simulink model "DS_distrIntp_1_10_simulated axes"  (R2019a)
settings: Solver=FixedStepDiscrete  StartTime=0.0  StopTime=inf  FixedStep=Ts  RelTol=1e-3
InitFcn:
  | %% Verwende vordefinierte Setpoints (Kreis mit Z-Komponente)
  | 
  | % Config
  | numCircles = 3;
  | scale=6;
  | %Versuch symmetrische Setpunkte zu setzen
  | pointsPerCircle =scale*(4+3*numCircles)+2;
  | 
  | r = 50;
  | m_x = r;
  | m_y = r;
  | 
  | % //
  | s = linspace(0,2*pi,pointsPerCircle);
  | 
  | setPoints_x = [];
  | setPoints_y = [];
  | 
  | for ii=1:numCircles
  | 
  | setPoints_x = [setPoints_x (-cos(s(1:floor(pointsPerCircle / 2))).*r + m_x + 2*r*(ii-1))]; %#ok<AGROW>
  | setPoints_y = [setPoints_y (sin(s).*r+m_y)]; %#ok<AGROW>pointsPerCircle / 2
  | 
  | end
  | 
  | setPoints_x = [setPoints_x flip(setPoints_x(1:end))];
  | 
  | % Loeschen doppelter y-Werte (Kreisuebergang)
  | setPoints_x(pointsPerCircle .* [1:numCircles]) = [];
  | setPoints_y(pointsPerCircle .* [1:numCircles]) = [];
  | 
  | % setPoints_x= [linspace(0,setPoints_x(19),19) setPoints_x(20:end)];
  | % setPoints_y= [linspace(0,setPoints_y(19),19) setPoints_y(20:end)];
  | 
  | % Array Elemente verschieben
  | % setPoints_x = circshift(setPoints_x,-pointsPerCircle/4,2);
  | % setPoints_y = circshift(setPoints_y,-pointsPerCircle/4,2);
  | 
  | z = zeros(1,size(setPoints_x,2));
  | z_x = -5:5;
  | z_y = -z_x.^2 + 25;
  | z_idx = 90;
  | z_idx2 = 210;
  | z(z_idx:z_idx+length(z_x)-1) = z_y;
  | z(z_idx2:z_idx2+length(z_x)-1) = z_y;
  | % z = [z_y z];
  | setPoints_z = z;
  | 
  | % setPoints_x = [zeros(1,length(z_y)) setPoints_x];
  | % setPoints_y = [setPoints_y(1,1)*ones(1,length(z_y)) setPoints_y];
  | 
  | % Umrechnung der Einheiten für Demonstrator
  | % setPoints_x = setPoints_x ./ 1000;
  | % setPoints_y = setPoints_y ./ 1000;
  | % setPoints_z = setPoints_z ./ 1000;
  | 
  | 
  | %{
  | plot(setPoints_x,setPoints_y);
  | fig = figure;
  | plot3(setPoints_x(1:end-1),setPoints_y(1:end-1),setPoints_z(1:end-1));
  | 
  | ax = gca;
  | ax.YDir = 'reverse';
  | ax.ZDir = 'reverse';
  | %}
  | 
  | % setPoints_z = zeros(1,size(setPoints_x,2));
  | 
  | setP_mat = [setPoints_x;setPoints_y;setPoints_z];
  | %Dauerlauftest zehn Durchgänge
  | %setP_mat = repmat(setP_mat, 1, 10);
  | setP_mat = setP_mat(:,2:end);
StartFcn:
  | close all;
model workspace (MAT data in the model file):
  MvmtPerfEval_collectVal = Simulink.Parameter
  MvmtPerfEval_collectVal.Value = 0.65
  MvmtPerfEval_collectVal.Description = '- Anteil eines Interpolationssegments (0,1)
    | - Nach Abarbeitung des spezifizierten Anteils wird gemeinsame Performance aller Agenten
    | vom Dispatcher geladen
    | 
    | - (!!!) Wert MUSS größer sein als MvmtPerfEval_sendOwnVal'
  MvmtPerfEval_collectVal.DataType = 'auto'
  MvmtPerfEval_collectVal.Min = 0
  MvmtPerfEval_collectVal.Max = 1
  MvmtPerfEval_collectVal.Dimensions = [1 1]
  MvmtPerfEval_sendOwnVal = Simulink.Parameter
  MvmtPerfEval_sendOwnVal.Value = 0.6
  MvmtPerfEval_sendOwnVal.Description = '- Anteil eines Interpolationssegments (0,1)
    | - Nach Abarbeitung des spezifizierten Anteils wird Perfomance Kennzahl an Dispatcher übermittelt
    | 
    | - (!!!) Wert MUSS kleiner sein als MvmtPerfEval_collectVal'
  MvmtPerfEval_sendOwnVal.DataType = 'auto'
  MvmtPerfEval_sendOwnVal.Min = 0
  MvmtPerfEval_sendOwnVal.Max = 1
  MvmtPerfEval_sendOwnVal.Dimensions = [1 1]
  PerfEval_numTicks_enable = Simulink.Parameter
  PerfEval_numTicks_enable.Value = 10
  PerfEval_numTicks_enable.Description = 'Anzahl der Ticks (Integrationsschritte), bevor die Performance ausgewertet wird
    | (unabhängig vom Senden des Werts an den Dispatcher)'
  PerfEval_numTicks_enable.DataType = 'auto'
  PerfEval_numTicks_enable.Dimensions = [1 1]
  Segmentregler_I_Gain = Simulink.Parameter
  Segmentregler_I_Gain.Value = 1
  Segmentregler_I_Gain.DataType = 'auto'
  Segmentregler_I_Gain.Dimensions = [1 1]
  Segmentregler_P_Gain = Simulink.Parameter
  Segmentregler_P_Gain.Value = 0
  Segmentregler_P_Gain.DataType = 'auto'
  Segmentregler_P_Gain.Dimensions = [1 1]
  Segmentregler_minVel_enable = Simulink.Parameter
  Segmentregler_minVel_enable.Value = 0.1
  Segmentregler_minVel_enable.DataType = 'auto'
  Segmentregler_minVel_enable.Dimensions = [1 1]
  Segmentregler_numTicks_enable = Simulink.Parameter
  Segmentregler_numTicks_enable.Value = 30
  Segmentregler_numTicks_enable.Description = 'Anzahl der Ticks (Integrationsschritte), bevor der Segmentregler aktiv wird'
  Segmentregler_numTicks_enable.DataType = 'auto'
  Segmentregler_numTicks_enable.Dimensions = [1 1]
  Ts = Simulink.Parameter
  Ts.Value = 0.005
  Ts.Description = 'Sampling Time'
  Ts.DataType = 'auto'
  Ts.Dimensions = [1 1]
  maxPos_x = Simulink.Parameter
  maxPos_x.Value = 300
  maxPos_x.Description = 'Grenze des Arbeitsbereichs (maximaler Wert der Koordinate)'
  maxPos_x.DataType = 'auto'
  maxPos_x.Dimensions = [1 1]
  maxPos_y = Simulink.Parameter
  maxPos_y.Value = 150
  maxPos_y.Description = 'Grenze des Arbeitsbereichs (maximaler Wert der Koordinate)'
  maxPos_y.DataType = 'auto'
  maxPos_y.Dimensions = [1 1]
  maxPos_z = Simulink.Parameter
  maxPos_z.Value = 50
  maxPos_z.Description = 'Grenze des Arbeitsbereichs (maximaler Wert der Koordinate)'
  maxPos_z.DataType = 'auto'
  maxPos_z.Dimensions = [1 1]
  maxVectorLengths = Simulink.Parameter
  maxVectorLengths.Value = 100000
  maxVectorLengths.DataType = 'auto'
  maxVectorLengths.Dimensions = [1 1]
  minAllowedVelSaturation = Simulink.Parameter
  minAllowedVelSaturation.Value = 0.05
  minAllowedVelSaturation.Description = 'Minimaler Saturation-Wert für den Geschwindigkeits-PID-Regler
    | (auch bei Sollgeschwindigkeit soll Fehlerkorrektur möglich sein)'
  minAllowedVelSaturation.DataType = 'auto'
  minAllowedVelSaturation.Dimensions = [1 1]
  numAxes = Simulink.Parameter
  numAxes.Value = 3
  numAxes.DataType = 'auto'
  numAxes.Dimensions = [1 1]
undefined symbols (not defined in the file or in its folder): DiscIntNeverNeededParam, VelOverride
libraries: simulink x19, vrlib x5, sldrtlib x2
(part 1 of 4)
settings Model: EnablePacing=on  PacingRate=10  Creator=Daniel  LastModifiedBy=Daniel
settings DataIOCC: ReturnWorkspaceOutputs=off
settings DebuggingCC: ArithmeticOperatorsInVariantConditions=warning

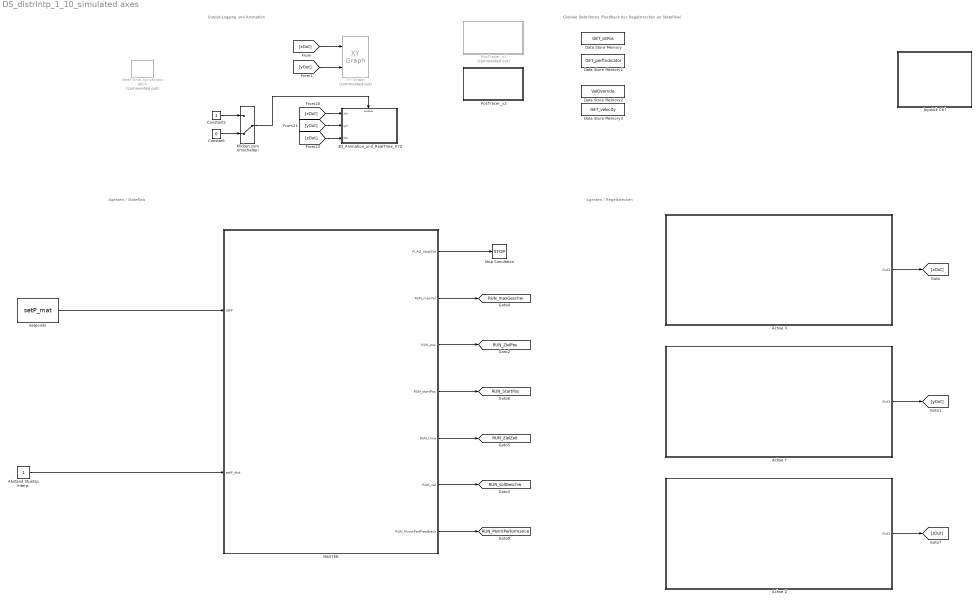
== system DS_distrIntp_1_10_simulated axes ==
  note: Globale DataStores (Feedback der Regelstrecken an Stateflow)
  note: Agenten / Regelstrecken
  note: Agenten / Stateflow
  note: Output-Logging und Animation
  3D_Animation_und_RealTime_XYZ : Subsystem
  Abstand Stuetzp. Interp. : Constant
  Achse X : Subsystem
  Achse Y : Subsystem
  Achse Z : Subsystem
  Constant : Constant  Value=0
  Constant1 : Constant
  Data Store Memory : DataStoreMemory  DataStoreName=GET_istPos  ReadBeforeWriteMsg=warning  WriteAfterWriteMsg=warning  WriteAfterReadMsg=warning  InitialValue=zeros(1,numAxes)  ShowAdditionalParam=off  OutDataTypeStr=double
  Data Store Memory1 : DataStoreMemory  DataStoreName=GET_perfIndicator  ReadBeforeWriteMsg=warning  WriteAfterWriteMsg=warning  WriteAfterReadMsg=warning  InitialValue=zeros(1,numAxes)  ShowAdditionalParam=off  OutDataTypeStr=double
  Data Store Memory2 : DataStoreMemory  DataStoreName=VelOverride  ReadBeforeWriteMsg=warning  WriteAfterWriteMsg=warning  WriteAfterReadMsg=warning  InitialValue=ones(1,numAxes)  ShowAdditionalParam=off  OutDataTypeStr=double
  Data Store Memory3 : DataStoreMemory  DataStoreName=GET_velocity  ReadBeforeWriteMsg=warning  WriteAfterWriteMsg=warning  WriteAfterReadMsg=warning  InitialValue=zeros(1,numAxes)  ShowAdditionalParam=off  OutDataTypeStr=double
  Joystick Ctrl : Subsystem
  Klicken zum Umschalten : ManualSwitch  CurrentSetting=0
  MASTER : Stateflow chart  TreatAsAtomicUnit=on
  PosTracer_v1 : Stateflow chart  Commented=on  BlockKeywords=__PRM__SERIALIZED__DATA__:Stateflow Chart,Stateflow Diagram  TreatAsAtomicUnit=on
  PosTracer_v2 : Stateflow chart  BlockKeywords=__PRM__SERIALIZED__DATA__:Stateflow Chart,Stateflow Diagram  TreatAsAtomicUnit=on
  Real-Time Synchronization : sldrtlib/Real-Time Synchronization  Commented=on  SampleTime=0.005  MaxMissedTicks=1000  ShowMissedTicks=off  YieldWhenWaiting=off
  Setpoints : Constant  Value=setP_mat
  Stop Simulation : Stop
  XY Graph : simulink/Sinks/XY Graph  Commented=on  xmin=0  xmax=maxPos_x  ymin=0  ymax=maxPos_y  st=-1
  tag scope: RUN_MvmtPerformance=global, RUN_StartPos=global, RUN_ZielPos=global, RUN_ZielZeit=global, RUN_maxGeschw=global, RUN_sollGeschw=global
  wires:
  Abstand Stuetzp. Interp./1 -> MASTER/2(setP_dist)
  Setpoints/1 -> MASTER/1(setP)
  Achse X/1(Out1) -> [xOut]
  [xOut] -> XY Graph/1
  [yOut] -> XY Graph/2
  Constant/1 -> Klicken zum Umschalten/2
  Constant1/1 -> Klicken zum Umschalten/1
  [xOut] -> 3D_Animation_und_RealTime_XYZ/1(xIn)
  [yOut] -> 3D_Animation_und_RealTime_XYZ/2(yIn)
  [zOut] -> 3D_Animation_und_RealTime_XYZ/3(zIn)
  MASTER/1(FLAG_stopSim) -> Stop Simulation/1
  MASTER/2(RUN_maxVel) -> [RUN_maxGeschw]
  MASTER/3(RUN_pos) -> [RUN_ZielPos]
  MASTER/4(RUN_startPos) -> [RUN_StartPos]
  MASTER/5(RUN_time) -> [RUN_ZielZeit]
  MASTER/6(RUN_vel) -> [RUN_sollGeschw]
  Achse Y/1(Out1) -> [yOut]
  Achse Z/1(Out1) -> [zOut]
  Klicken zum Umschalten/1 -> 3D_Animation_und_RealTime_XYZ/Enable
  MASTER/7(RUN_MvmtPerfFeedback) -> [RUN_MvmtPerformance]

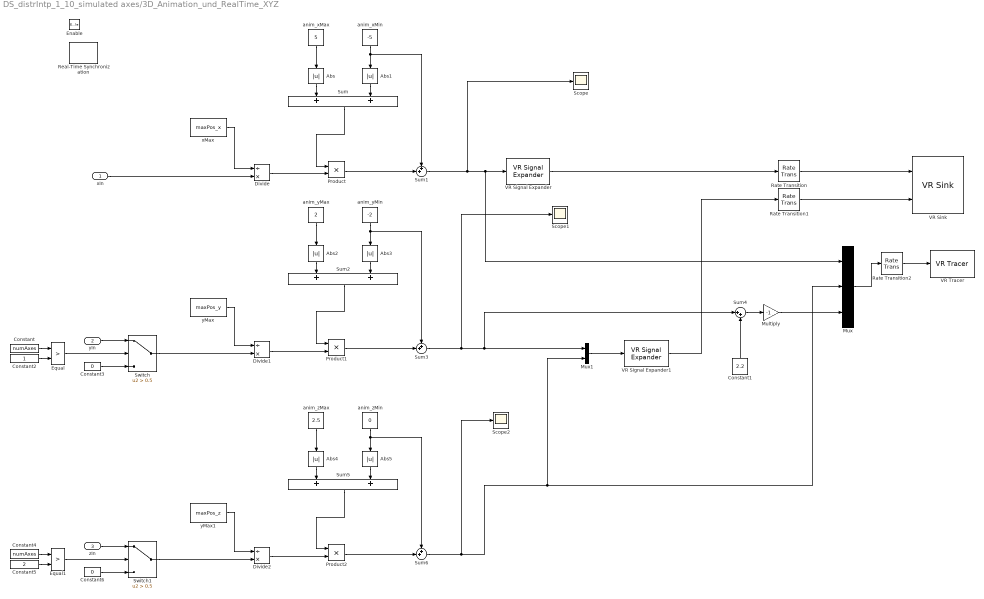
== system DS_distrIntp_1_10_simulated axes/3D_Animation_und_RealTime_XYZ ==
  xIn : Inport
  yIn : Inport  Port=2
  zIn : Inport  Port=3
  Enable : EnablePort
  Abs{,1..5} (6 alike) : Abs
  Constant : Constant  Value=numAxes
  Constant1 : Constant  Value=2.2
  Constant2 : Constant
  Constant3 : Constant  Value=0
  Constant4 : Constant  Value=numAxes
  Constant5 : Constant  Value=2
  Constant6 : Constant  Value=0
  Divide : Product  Inputs=/*
  Divide1 : Product  Inputs=/*
  Divide2 : Product  Inputs=/*
  Equal : RelationalOperator  Operator=>  OutDataTypeStr=boolean  RndMeth=Simplest
  Equal1 : RelationalOperator  Operator=>  OutDataTypeStr=boolean  RndMeth=Simplest
  Multiply : Gain  Gain=-1
  Mux : Mux  Inputs=3
  Mux1 : Mux  Inputs=2
  Product : Product
  Product1 : Product
  Product2 : Product
  Rate Transition : RateTransition  OutPortSampleTime=0.1
  Rate Transition1 : RateTransition  OutPortSampleTime=0.1
  Rate Transition2 : RateTransition  OutPortSampleTime=0.3
  Real-Time Synchronization : sldrtlib/Real-Time Synchronization  SampleTime=0.005  MaxMissedTicks=1000  ShowMissedTicks=off  YieldWhenWaiting=off
  Scope : Scope
  Scope1 : Scope
  Scope2 : Scope
  Sum : Sum
  Sum1 : Sum  Inputs=++|
  Sum2 : Sum
  Sum3 : Sum  Inputs=++|
  Sum4 : Sum  Inputs=|++
  Sum5 : Sum
  Sum6 : Sum  Inputs=++|
  Switch : Switch  Criteria=u2 > Threshold  Threshold=0.5
  Switch1 : Switch  Criteria=u2 > Threshold  Threshold=0.5
  VR Signal Expander : vrlib/VR Signal Expander  outwidth=3  outidx=1
      settings: SourceProductName=Simulink
  VR Signal Expander1 : vrlib/VR Signal Expander  outwidth=3  outidx=[1 2]
      settings: SourceProductName=Simulink
  VR Sink : vrlib/VR Sink  InstantiateOnLoad=on  SampleTime=-1  ViewEnable=on  RemoteChange=off  RemoteView=off  FieldsWritten=yAchse.translation.3.1.1.double#TCP.translation.3.1.1.double  WorldFileName=DS_MA_3dworld.wrl  WorldDescription=DS_MA_3dworld  AutoView=on  VideoDimensions=[]  AllowVariableSize=off  FigureProperties="{'Position', 'Name', 'Viewpoint', 'CameraBound', 'CameraDirection', 'CameraPosition', 'CameraUpVector', 'ZoomFactor', 'Antialiasing', 'Headlight', 'Lighting', 'NavPanel', 'Sound', 'StatusBar', 'Stereo3D', 'Stereo3DCameraOffset', 'Stereo3DHIT', 'ToolBar', 'Textures', 'Transparency', 'Triad', 'Wireframe', 'NavZones', 'NavMode', 'NavSpeed', 'CaptureFileFormat', 'CaptureFileName', 'Record2DCompressMethod', 'Record2DCompressQuality', 'Record2D', 'Record2DFileName', 'Record2DFPS'; [5.0000000000000000e+00   9.2000000000000000e+01   5.7600000000000000e+02   3.5000000000000000e+02], 'DS_MA_3dworld', '_untitled_1', 'on', [0.0000000000000000e+00   0.0000000000000000e+00  -1.0000000000000000e+00], [0.0000000000000000e+00   0.0000000000000000e+00   0.0000000000000000e+00], [0.0000000000000000e+00   1.0000000000000000e+00   0.0000000000000000e+00], [1.0000000000000000e+00], 'on', 'on', 'on', 'halfbar', 'on', 'on', 'off', [1.0000000149011612e-01], [0.0000000000000000e+00], 'on', 'on', 'on', 'none', 'off', 'off', 'fly', 'normal', 'tif', '%f_anim_%n.tif', 'auto', [7.5000000000000000e+01], 'off', '%f_anim_%n.avi', 'auto'}"
      settings: SourceProductName=Simulink
  VR Tracer : vrlib/VR Tracer  VrmlFile=DS_MA_3dworld.wrl  MarkerName=Tetrahedron  UseLines=on  UseTriads=on  MarkerScale=[0.1 0.1 0.1]  MarkerColorSelection=Selected from color list  MarkerColor=red  rgbval=[1 0 0]  Ts=0.3  ForceViewerOpen=off  ConnectPlane=off  PlaneCoeff=[0 1 0 0]  ConnectPoint=None  PointCoord=[0 0 0]
      settings: SourceProductName=Simulink  SourceProductBaseCode=SL
  anim_xMax : Constant  Value=5
  anim_xMin : Constant  Value=-5
  anim_yMax : Constant  Value=2
  anim_yMin : Constant  Value=-2
  anim_zMax : Constant  Value=2.5
  anim_zMin : Constant  Value=0
  xMax : Constant  Value=maxPos_x
  yMax : Constant  Value=maxPos_y
  yMax1 : Constant  Value=maxPos_z
  wires:
  Constant1/1 -> Sum4/2
  Sum4/1 -> Multiply/1
  Multiply/1 -> Mux/3
  Rate Transition2/1 -> VR Tracer/1
  Mux/1 -> Rate Transition2/1
  Rate Transition1/1 -> VR Sink/2
  Rate Transition/1 -> VR Sink/1
  VR Signal Expander/1 -> Rate Transition/1
  VR Signal Expander1/1 -> Rate Transition1/1
  Sum3/1 -> Mux1/1, Sum4/1, Scope1/1
  Sum1/1 -> VR Signal Expander/1, Mux/1, Scope/1
  Switch/1 -> Divide1/2
  yMax/1 -> Divide1/1
  anim_yMax/1 -> Abs2/1
  anim_yMin/1 -> Sum3/1, Abs3/1
  Abs2/1 -> Sum2/1
  Abs3/1 -> Sum2/2
  Divide1/1 -> Product1/2
  Sum2/1 -> Product1/1
  Product1/1 -> Sum3/2
  Product/1 -> Sum1/2
  Sum/1 -> Product/1
  Divide/1 -> Product/2
  Abs1/1 -> Sum/2
  Abs/1 -> Sum/1
  anim_xMin/1 -> Abs1/1, Sum1/1
  anim_xMax/1 -> Abs/1
  xMax/1 -> Divide/1
  xIn/1 -> Divide/2
  Product2/1 -> Sum6/2
  Sum5/1 -> Product2/1
  Divide2/1 -> Product2/2
  Abs5/1 -> Sum5/2
  Abs4/1 -> Sum5/1
  anim_zMin/1 -> Abs5/1, Sum6/1
  anim_zMax/1 -> Abs4/1
  yMax1/1 -> Divide2/1
  Switch1/1 -> Divide2/2
  Sum6/1 -> Scope2/1, Mux1/2, Mux/2
  Mux1/1 -> VR Signal Expander1/1
  Constant/1 -> Equal/1
  Constant2/1 -> Equal/2
  yIn/1 -> Switch/1
  Equal/1 -> Switch/2
  Constant3/1 -> Switch/3
  Constant6/1 -> Switch1/3
  Equal1/1 -> Switch1/2
  zIn/1 -> Switch1/1
  Constant5/1 -> Equal1/2
  Constant4/1 -> Equal1/1

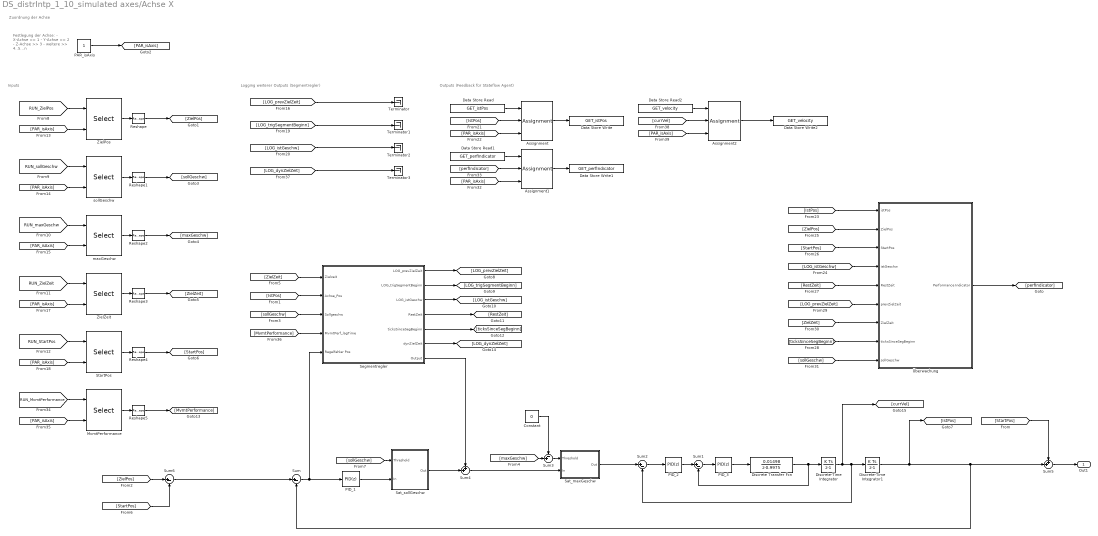
== system DS_distrIntp_1_10_simulated axes/Achse X ==
  note: Outputs (Feedback für Stateflow Agent)
  note: Logging weiterer Outputs (Segmentregler)
  note: Zuordnung der Achse
  note: Festlegung der Achse:
      | - X-Achse >> 1
      | - Y-Achse >> 2
      | - Z-Achse >> 3
      | - weitere >> 4..5...n
  note: Inputs
  Assignment : Assignment  DiagnosticForDimensions=Warning  IndexOptions=Index vector (port)  Indices=1  OutputSizes=1
  Assignment1 : Assignment  DiagnosticForDimensions=Warning  IndexOptions=Index vector (port)  Indices=1  OutputSizes=1
  Assignment2 : Assignment  DiagnosticForDimensions=Warning  IndexOptions=Index vector (port)  Indices=1  OutputSizes=1
  Constant : Constant  Value=0
  Data Store Read : DataStoreRead  DataStoreName=GET_istPos
  Data Store Read1 : DataStoreRead  DataStoreName=GET_perfIndicator
  Data Store Read2 : DataStoreRead  DataStoreName=GET_velocity
  Data Store Write : DataStoreWrite  DataStoreName=GET_istPos
  Data Store Write1 : DataStoreWrite  DataStoreName=GET_perfIndicator
  Data Store Write2 : DataStoreWrite  DataStoreName=GET_velocity
  Discrete Transfer Fcn : DiscreteTransferFcn  Numerator=0.01498  Denominator=[1 -0.9975]
  Discrete-Time Integrator : DiscreteIntegrator  SampleTime=-1  ICPrevOutput=DiscIntNeverNeededParam  ICPrevScaledInput=DiscIntNeverNeededParam
  Discrete-Time Integrator1 : DiscreteIntegrator  SampleTime=-1  ICPrevOutput=DiscIntNeverNeededParam  ICPrevScaledInput=DiscIntNeverNeededParam
  MvmtPerformance : Selector  IndexOptions=Index vector (port)  Indices=[1 3]  OutputSizes=1
  PAR_isAxis : Constant
  PID_1 : simulink/Continuous/PID Controller  Controller=PID  Form=Parallel  TimeDomain=Discrete-time  SampleTime=-1  IntegratorMethod=Forward Euler  FilterMethod=Forward Euler  ControllerParametersSource=internal  P=20  I=0  D=0  UseFilter=on  N=100  TunerSelectOption=Transfer Function Based (PID Tuner App)  InitialConditionSource=internal  InitialConditionForIntegrator=0  InitialConditionForFilter=0  DifferentiatorICPrevScaledInput=0  ExternalReset=none  TrackingMode=off  Kt=1  LimitOutput=off  UpperSaturationLimit=inf  LowerSaturationLimit=-inf  LinearizeAsGain=off  AntiWindupMode=none  Kb=1  POutMin=[]  POutMax=[]  IOutMin=[]  IOutMax=[]  DOutMin=[]  DOutMax=[]  NOutMin=[]  NOutMax=[]  SumOutMin=[]  SumOutMax=[]  SaturationOutMin=[]  SaturationOutMax=[]  PParamMin=[]  PParamMax=[]  IParamMin=[]  IParamMax=[]  DParamMin=[]  DParamMax=[]  NParamMin=[]  NParamMax=[]  KbParamMin=[]  KbParamMax=[]  KtParamMin=[]  KtParamMax=[]  KbOutMin=[]  KbOutMax=[]  KtOutMin=[]  KtOutMax=[]  IntegratorOutMin=[]  IntegratorOutMax=[]  FilterOutMin=[]  FilterOutMax=[]  SumI1OutMin=[]  SumI1OutMax=[]  SumI2OutMin=[]  SumI2OutMax=[]  SumI3OutMin=[]  SumI3OutMax=[]  SumI4OutMin=[]  SumI4OutMax=[]  SumDOutMin=[]  SumDOutMax=[]  DifferentiatorOutMin=[]  DifferentiatorOutMax=[]  FilterDiffOutCoefMin=[]  FilterDiffOutCoefMax=[]  ReciprocalOutMin=[]  ReciprocalOutMax=[]  SumDenOutMin=[]  SumDenOutMax=[]  SumNumOutMin=[]  SumNumOutMax=[]  DivideOutMin=[]  DivideOutMax=[]  IntegratorContinuousStateAttributes=''  IntegratorStateMustResolveToSignalObject=off  IntegratorRTWStateStorageClass=Auto  FilterContinuousStateAttributes=''  FilterStateMustResolveToSignalObject=off  FilterRTWStateStorageClass=Auto  ParallelPVariant=InternalParameters  IdealPVariant=Disabled  IVariant=InternalParameters  DVariant=InternalParameters  IntegratorVariant=Discrete  SatVariant=Disabled  AWVariant=Passthrough  PCopyVariant=Disabled  TRVariant=Disabled  FdbkBlocksVariant=Forward  IdealPFdbkVariant=Disabled  SatFdbkVariant=Disabled  DerivativeFilterVariant=ForwardEulerFilter  NVariant=InternalParameters  NCopyVariant=Disabled  FilterICVariant=InternalICsFilter  IntegratorICVariant=InternalICs  ExternalResetVariant=Disabled  TRSumVariant=Passthrough  SumFdbkVariant=Disabled  SumVariant=Sum_PID
  PID_2 : simulink/Continuous/PID Controller  Controller=PID  Form=Parallel  TimeDomain=Discrete-time  SampleTime=-1  IntegratorMethod=Forward Euler  FilterMethod=Forward Euler  ControllerParametersSource=internal  P=20  I=1  D=0  UseFilter=on  N=100  TunerSelectOption=Transfer Function Based (PID Tuner App)  InitialConditionSource=internal  InitialConditionForIntegrator=0  InitialConditionForFilter=0  DifferentiatorICPrevScaledInput=0  ExternalReset=none  TrackingMode=off  Kt=1  LimitOutput=off  UpperSaturationLimit=inf  LowerSaturationLimit=-inf  LinearizeAsGain=off  AntiWindupMode=none  Kb=1  POutMin=[]  POutMax=[]  IOutMin=[]  IOutMax=[]  DOutMin=[]  DOutMax=[]  NOutMin=[]  NOutMax=[]  SumOutMin=[]  SumOutMax=[]  SaturationOutMin=[]  SaturationOutMax=[]  PParamMin=[]  PParamMax=[]  IParamMin=[]  IParamMax=[]  DParamMin=[]  DParamMax=[]  NParamMin=[]  NParamMax=[]  KbParamMin=[]  KbParamMax=[]  KtParamMin=[]  KtParamMax=[]  KbOutMin=[]  KbOutMax=[]  KtOutMin=[]  KtOutMax=[]  IntegratorOutMin=[]  IntegratorOutMax=[]  FilterOutMin=[]  FilterOutMax=[]  SumI1OutMin=[]  SumI1OutMax=[]  SumI2OutMin=[]  SumI2OutMax=[]  SumI3OutMin=[]  SumI3OutMax=[]  SumI4OutMin=[]  SumI4OutMax=[]  SumDOutMin=[]  SumDOutMax=[]  DifferentiatorOutMin=[]  DifferentiatorOutMax=[]  FilterDiffOutCoefMin=[]  FilterDiffOutCoefMax=[]  ReciprocalOutMin=[]  ReciprocalOutMax=[]  SumDenOutMin=[]  SumDenOutMax=[]  SumNumOutMin=[]  SumNumOutMax=[]  DivideOutMin=[]  DivideOutMax=[]  IntegratorContinuousStateAttributes=''  IntegratorStateMustResolveToSignalObject=off  IntegratorRTWStateStorageClass=Auto  FilterContinuousStateAttributes=''  FilterStateMustResolveToSignalObject=off  FilterRTWStateStorageClass=Auto  ParallelPVariant=InternalParameters  IdealPVariant=Disabled  IVariant=InternalParameters  DVariant=InternalParameters  IntegratorVariant=Discrete  SatVariant=Disabled  AWVariant=Passthrough  PCopyVariant=Disabled  TRVariant=Disabled  FdbkBlocksVariant=Forward  IdealPFdbkVariant=Disabled  SatFdbkVariant=Disabled  DerivativeFilterVariant=ForwardEulerFilter  NVariant=InternalParameters  NCopyVariant=Disabled  FilterICVariant=InternalICsFilter  IntegratorICVariant=InternalICs  ExternalResetVariant=Disabled  TRSumVariant=Passthrough  SumFdbkVariant=Disabled  SumVariant=Sum_PID
  PID_3 : simulink/Continuous/PID Controller  Controller=PID  Form=Parallel  TimeDomain=Discrete-time  SampleTime=-1  IntegratorMethod=Forward Euler  FilterMethod=Forward Euler  ControllerParametersSource=internal  P=20  I=1  D=0  UseFilter=on  N=100  TunerSelectOption=Transfer Function Based (PID Tuner App)  InitialConditionSource=internal  InitialConditionForIntegrator=0  InitialConditionForFilter=0  DifferentiatorICPrevScaledInput=0  ExternalReset=none  TrackingMode=off  Kt=1  LimitOutput=off  UpperSaturationLimit=inf  LowerSaturationLimit=-inf  LinearizeAsGain=off  AntiWindupMode=none  Kb=1  POutMin=[]  POutMax=[]  IOutMin=[]  IOutMax=[]  DOutMin=[]  DOutMax=[]  NOutMin=[]  NOutMax=[]  SumOutMin=[]  SumOutMax=[]  SaturationOutMin=[]  SaturationOutMax=[]  PParamMin=[]  PParamMax=[]  IParamMin=[]  IParamMax=[]  DParamMin=[]  DParamMax=[]  NParamMin=[]  NParamMax=[]  KbParamMin=[]  KbParamMax=[]  KtParamMin=[]  KtParamMax=[]  KbOutMin=[]  KbOutMax=[]  KtOutMin=[]  KtOutMax=[]  IntegratorOutMin=[]  IntegratorOutMax=[]  FilterOutMin=[]  FilterOutMax=[]  SumI1OutMin=[]  SumI1OutMax=[]  SumI2OutMin=[]  SumI2OutMax=[]  SumI3OutMin=[]  SumI3OutMax=[]  SumI4OutMin=[]  SumI4OutMax=[]  SumDOutMin=[]  SumDOutMax=[]  DifferentiatorOutMin=[]  DifferentiatorOutMax=[]  FilterDiffOutCoefMin=[]  FilterDiffOutCoefMax=[]  ReciprocalOutMin=[]  ReciprocalOutMax=[]  SumDenOutMin=[]  SumDenOutMax=[]  SumNumOutMin=[]  SumNumOutMax=[]  DivideOutMin=[]  DivideOutMax=[]  IntegratorContinuousStateAttributes=''  IntegratorStateMustResolveToSignalObject=off  IntegratorRTWStateStorageClass=Auto  FilterContinuousStateAttributes=''  FilterStateMustResolveToSignalObject=off  FilterRTWStateStorageClass=Auto  ParallelPVariant=InternalParameters  IdealPVariant=Disabled  IVariant=InternalParameters  DVariant=InternalParameters  IntegratorVariant=Discrete  SatVariant=Disabled  AWVariant=Passthrough  PCopyVariant=Disabled  TRVariant=Disabled  FdbkBlocksVariant=Forward  IdealPFdbkVariant=Disabled  SatFdbkVariant=Disabled  DerivativeFilterVariant=ForwardEulerFilter  NVariant=InternalParameters  NCopyVariant=Disabled  FilterICVariant=InternalICsFilter  IntegratorICVariant=InternalICs  ExternalResetVariant=Disabled  TRSumVariant=Passthrough  SumFdbkVariant=Disabled  SumVariant=Sum_PID
  Reshape{,1..5} (6 alike) : Reshape
  Sat_maxGeschw : Subsystem
  Sat_sollGeschw : Subsystem
  Segmentregler : Subsystem
  StartPos : Selector  IndexOptions=Index vector (port)  Indices=[1 3]  OutputSizes=1
  Sum{,1..2,6} (4 alike) : Sum  Inputs=|+-
  Sum3 : Sum  Inputs=-+|
  Sum4 : Sum  Inputs=++|
  Sum5 : Sum  Inputs=++|
  Terminator{,1..3} (4 alike) : Terminator
  ZielPos : Selector  IndexOptions=Index vector (port)  Indices=[1 3]  OutputSizes=1
  ZielZeit : Selector  IndexOptions=Index vector (port)  Indices=[1 3]  OutputSizes=1
  maxGeschw : Selector  IndexOptions=Index vector (port)  Indices=[1 3]  OutputSizes=1
  sollGeschw : Selector  IndexOptions=Index vector (port)  Indices=[1 3]  OutputSizes=1
  Überwachung : Subsystem
  Out1 : Outport  VectorParamsAs1DForOutWhenUnconnected=off
  wires:
  Sum/1 -> Segmentregler/5(Regelfehler Pos), PID_1/1
  PID_1/1 -> Sat_sollGeschw/2(In)
  Sat_sollGeschw/1(Out) -> Sum4/2
  Sum4/1 -> Sat_maxGeschw/2(In)
  PID_3/1 -> Discrete Transfer Fcn/1
  Discrete Transfer Fcn/1 -> Discrete-Time Integrator/1, Sum1/2
  Sum2/1 -> PID_2/1
  Sum6/1 -> Sum/1
  Discrete-Time Integrator/1 -> [currVel], Discrete-Time Integrator1/1, Sum2/2
  Sum1/1 -> PID_3/1
  PID_2/1 -> Sum1/1
  Sat_maxGeschw/1(Out) -> Sum2/1
  Discrete-Time Integrator1/1 -> [IstPos], Sum5/2, Sum/2
  Sum5/1 -> Out1/1
  [ZielPos] -> Sum6/1
  [ZielZeit] -> Segmentregler/1(Zielzeit)
  [IstPos] -> Segmentregler/2(Achse_Pos)
  Segmentregler/7(Output) -> Sum4/1
  [StartPos] -> Sum5/1
  [StartPos] -> Sum6/2
  [sollGeschw] -> Segmentregler/3(Sollgeschw)
  [sollGeschw] -> Sat_sollGeschw/1(Threshold)
  PAR_isAxis/1 -> [PAR_isAxis]
  [PAR_isAxis] -> ZielPos/2
  [RUN_ZielPos] -> ZielPos/1
  ZielPos/1 -> Reshape/1
  sollGeschw/1 -> Reshape1/1
  [RUN_sollGeschw] -> sollGeschw/1
  [PAR_isAxis] -> sollGeschw/2
  [PAR_isAxis] -> maxGeschw/2
  [RUN_maxGeschw] -> maxGeschw/1
  maxGeschw/1 -> Reshape2/1
  ZielZeit/1 -> Reshape3/1
  [RUN_ZielZeit] -> ZielZeit/1
  [PAR_isAxis] -> ZielZeit/2
  [PAR_isAxis] -> StartPos/2
  [RUN_StartPos] -> StartPos/1
  StartPos/1 -> Reshape4/1
  Segmentregler/1(LOG_prevZielZeit) -> [LOG_prevZielZeit]
  Segmentregler/2(LOG_trigSegmentBeginn) -> [LOG_trigSegmentBeginn]
  Segmentregler/3(LOG_istGeschw) -> [LOG_istGeschw]
  [LOG_prevZielZeit] -> Terminator/1
  [LOG_trigSegmentBeginn] -> Terminator1/1
  Reshape/1 -> [ZielPos]
  Reshape1/1 -> [sollGeschw]
  Reshape2/1 -> [maxGeschw]
  Reshape4/1 -> [StartPos]
  Reshape3/1 -> [ZielZeit]
  Data Store Read/1 -> Assignment/1
  [IstPos] -> Assignment/2
  [PAR_isAxis] -> Assignment/3
  Assignment/1 -> Data Store Write/1
  Segmentregler/4(RestZeit) -> [RestZeit]
  [maxGeschw] -> Sum3/2
  Sum3/1 -> Sat_maxGeschw/1(Threshold)
  Constant/1 -> Sum3/1
  [IstPos] -> Überwachung/1(istPos)
  [ZielPos] -> Überwachung/2(ZielPos)
  [StartPos] -> Überwachung/3(StartPos)
  [LOG_istGeschw] -> Überwachung/4(istGeschw)
  [RestZeit] -> Überwachung/5(RestZeit)
  [LOG_prevZielZeit] -> Überwachung/6(prevZielZeit)
  [ZielZeit] -> Überwachung/7(ZielZeit)
  Assignment1/1 -> Data Store Write1/1
  [PAR_isAxis] -> Assignment1/3
  [perfIndicator] -> Assignment1/2
  Data Store Read1/1 -> Assignment1/1
  Überwachung/1(Performance Indicator) -> [perfIndicator]
  Segmentregler/5(ticksSinceSegBeginn) -> [ticksSinceSegBeginn]
  [ticksSinceSegBeginn] -> Überwachung/8(ticksSinceSegBeginn)
  [sollGeschw] -> Überwachung/9(sollGeschw)
  Reshape5/1 -> [MvmtPerformance]
  MvmtPerformance/1 -> Reshape5/1
  [RUN_MvmtPerformance] -> MvmtPerformance/1
  [PAR_isAxis] -> MvmtPerformance/2
  [MvmtPerformance] -> Segmentregler/4(MvmtPerf_lagTime)
  Segmentregler/6(dynZielZeit) -> [LOG_dynZielZeit]
  [LOG_dynZielZeit] -> Terminator3/1
  [PAR_isAxis] -> Assignment2/3
  [currVel] -> Assignment2/2
  Data Store Read2/1 -> Assignment2/1
  Assignment2/1 -> Data Store Write2/1
  [LOG_istGeschw] -> Terminator2/1

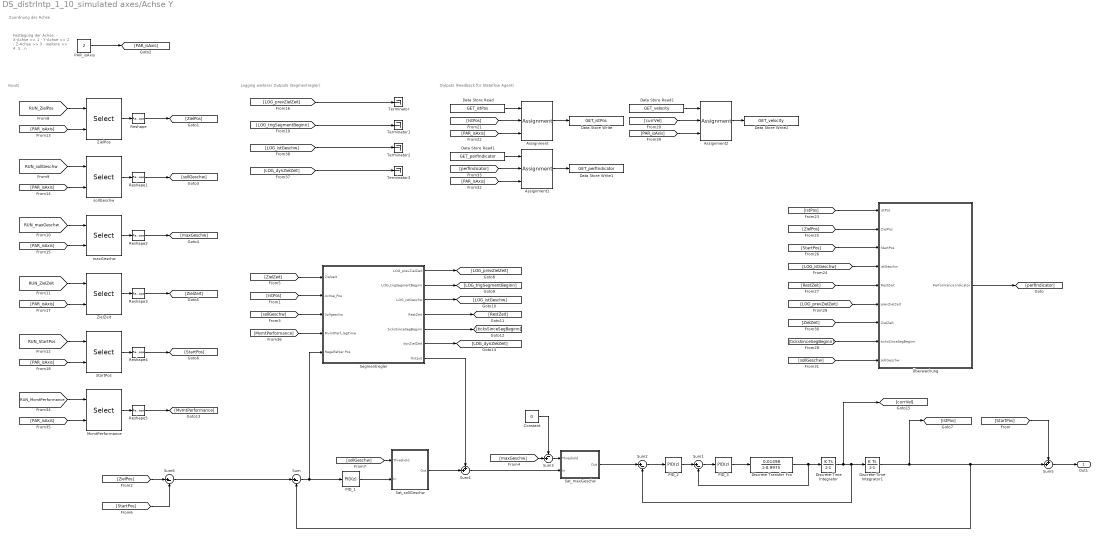
== system DS_distrIntp_1_10_simulated axes/Achse Y ==
  note: Inputs
  note: Festlegung der Achse:
      | - X-Achse >> 1
      | - Y-Achse >> 2
      | - Z-Achse >> 3
      | - weitere >> 4..5...n
  note: Zuordnung der Achse
  note: Logging weiterer Outputs (Segmentregler)
  note: Outputs (Feedback für Stateflow Agent)
  Assignment : Assignment  DiagnosticForDimensions=Warning  IndexOptions=Index vector (port)  Indices=1  OutputSizes=1
  Assignment1 : Assignment  DiagnosticForDimensions=Warning  IndexOptions=Index vector (port)  Indices=1  OutputSizes=1
  Assignment2 : Assignment  DiagnosticForDimensions=Warning  IndexOptions=Index vector (port)  Indices=1  OutputSizes=1
  Constant : Constant  Value=0
  Data Store Read : DataStoreRead  DataStoreName=GET_istPos
  Data Store Read1 : DataStoreRead  DataStoreName=GET_perfIndicator
  Data Store Read2 : DataStoreRead  DataStoreName=GET_velocity
  Data Store Write : DataStoreWrite  DataStoreName=GET_istPos
  Data Store Write1 : DataStoreWrite  DataStoreName=GET_perfIndicator
  Data Store Write2 : DataStoreWrite  DataStoreName=GET_velocity
  Discrete Transfer Fcn : DiscreteTransferFcn  Numerator=0.01498  Denominator=[1 -0.9975]
  Discrete-Time Integrator : DiscreteIntegrator  SampleTime=-1  ICPrevOutput=DiscIntNeverNeededParam  ICPrevScaledInput=DiscIntNeverNeededParam
  Discrete-Time Integrator1 : DiscreteIntegrator  SampleTime=-1  ICPrevOutput=DiscIntNeverNeededParam  ICPrevScaledInput=DiscIntNeverNeededParam
  MvmtPerformance : Selector  IndexOptions=Index vector (port)  Indices=[1 3]  OutputSizes=1
  PAR_isAxis : Constant  Value=2
  PID_1 : simulink/Continuous/PID Controller  Controller=PID  Form=Parallel  TimeDomain=Discrete-time  SampleTime=-1  IntegratorMethod=Forward Euler  FilterMethod=Forward Euler  ControllerParametersSource=internal  P=20  I=0  D=0  UseFilter=on  N=100  TunerSelectOption=Transfer Function Based (PID Tuner App)  InitialConditionSource=internal  InitialConditionForIntegrator=0  InitialConditionForFilter=0  DifferentiatorICPrevScaledInput=0  ExternalReset=none  TrackingMode=off  Kt=1  LimitOutput=off  UpperSaturationLimit=inf  LowerSaturationLimit=-inf  LinearizeAsGain=off  AntiWindupMode=none  Kb=1  POutMin=[]  POutMax=[]  IOutMin=[]  IOutMax=[]  DOutMin=[]  DOutMax=[]  NOutMin=[]  NOutMax=[]  SumOutMin=[]  SumOutMax=[]  SaturationOutMin=[]  SaturationOutMax=[]  PParamMin=[]  PParamMax=[]  IParamMin=[]  IParamMax=[]  DParamMin=[]  DParamMax=[]  NParamMin=[]  NParamMax=[]  KbParamMin=[]  KbParamMax=[]  KtParamMin=[]  KtParamMax=[]  KbOutMin=[]  KbOutMax=[]  KtOutMin=[]  KtOutMax=[]  IntegratorOutMin=[]  IntegratorOutMax=[]  FilterOutMin=[]  FilterOutMax=[]  SumI1OutMin=[]  SumI1OutMax=[]  SumI2OutMin=[]  SumI2OutMax=[]  SumI3OutMin=[]  SumI3OutMax=[]  SumI4OutMin=[]  SumI4OutMax=[]  SumDOutMin=[]  SumDOutMax=[]  DifferentiatorOutMin=[]  DifferentiatorOutMax=[]  FilterDiffOutCoefMin=[]  FilterDiffOutCoefMax=[]  ReciprocalOutMin=[]  ReciprocalOutMax=[]  SumDenOutMin=[]  SumDenOutMax=[]  SumNumOutMin=[]  SumNumOutMax=[]  DivideOutMin=[]  DivideOutMax=[]  IntegratorContinuousStateAttributes=''  IntegratorStateMustResolveToSignalObject=off  IntegratorRTWStateStorageClass=Auto  FilterContinuousStateAttributes=''  FilterStateMustResolveToSignalObject=off  FilterRTWStateStorageClass=Auto  ParallelPVariant=InternalParameters  IdealPVariant=Disabled  IVariant=InternalParameters  DVariant=InternalParameters  IntegratorVariant=Discrete  SatVariant=Disabled  AWVariant=Passthrough  PCopyVariant=Disabled  TRVariant=Disabled  FdbkBlocksVariant=Forward  IdealPFdbkVariant=Disabled  SatFdbkVariant=Disabled  DerivativeFilterVariant=ForwardEulerFilter  NVariant=InternalParameters  NCopyVariant=Disabled  FilterICVariant=InternalICsFilter  IntegratorICVariant=InternalICs  ExternalResetVariant=Disabled  TRSumVariant=Passthrough  SumFdbkVariant=Disabled  SumVariant=Sum_PID
  PID_2 : simulink/Continuous/PID Controller  Controller=PID  Form=Parallel  TimeDomain=Discrete-time  SampleTime=-1  IntegratorMethod=Forward Euler  FilterMethod=Forward Euler  ControllerParametersSource=internal  P=20  I=1  D=0  UseFilter=on  N=100  TunerSelectOption=Transfer Function Based (PID Tuner App)  InitialConditionSource=internal  InitialConditionForIntegrator=0  InitialConditionForFilter=0  DifferentiatorICPrevScaledInput=0  ExternalReset=none  TrackingMode=off  Kt=1  LimitOutput=off  UpperSaturationLimit=inf  LowerSaturationLimit=-inf  LinearizeAsGain=off  AntiWindupMode=none  Kb=1  POutMin=[]  POutMax=[]  IOutMin=[]  IOutMax=[]  DOutMin=[]  DOutMax=[]  NOutMin=[]  NOutMax=[]  SumOutMin=[]  SumOutMax=[]  SaturationOutMin=[]  SaturationOutMax=[]  PParamMin=[]  PParamMax=[]  IParamMin=[]  IParamMax=[]  DParamMin=[]  DParamMax=[]  NParamMin=[]  NParamMax=[]  KbParamMin=[]  KbParamMax=[]  KtParamMin=[]  KtParamMax=[]  KbOutMin=[]  KbOutMax=[]  KtOutMin=[]  KtOutMax=[]  IntegratorOutMin=[]  IntegratorOutMax=[]  FilterOutMin=[]  FilterOutMax=[]  SumI1OutMin=[]  SumI1OutMax=[]  SumI2OutMin=[]  SumI2OutMax=[]  SumI3OutMin=[]  SumI3OutMax=[]  SumI4OutMin=[]  SumI4OutMax=[]  SumDOutMin=[]  SumDOutMax=[]  DifferentiatorOutMin=[]  DifferentiatorOutMax=[]  FilterDiffOutCoefMin=[]  FilterDiffOutCoefMax=[]  ReciprocalOutMin=[]  ReciprocalOutMax=[]  SumDenOutMin=[]  SumDenOutMax=[]  SumNumOutMin=[]  SumNumOutMax=[]  DivideOutMin=[]  DivideOutMax=[]  IntegratorContinuousStateAttributes=''  IntegratorStateMustResolveToSignalObject=off  IntegratorRTWStateStorageClass=Auto  FilterContinuousStateAttributes=''  FilterStateMustResolveToSignalObject=off  FilterRTWStateStorageClass=Auto  ParallelPVariant=InternalParameters  IdealPVariant=Disabled  IVariant=InternalParameters  DVariant=InternalParameters  IntegratorVariant=Discrete  SatVariant=Disabled  AWVariant=Passthrough  PCopyVariant=Disabled  TRVariant=Disabled  FdbkBlocksVariant=Forward  IdealPFdbkVariant=Disabled  SatFdbkVariant=Disabled  DerivativeFilterVariant=ForwardEulerFilter  NVariant=InternalParameters  NCopyVariant=Disabled  FilterICVariant=InternalICsFilter  IntegratorICVariant=InternalICs  ExternalResetVariant=Disabled  TRSumVariant=Passthrough  SumFdbkVariant=Disabled  SumVariant=Sum_PID
  PID_3 : simulink/Continuous/PID Controller  Controller=PID  Form=Parallel  TimeDomain=Discrete-time  SampleTime=-1  IntegratorMethod=Forward Euler  FilterMethod=Forward Euler  ControllerParametersSource=internal  P=20  I=1  D=0  UseFilter=on  N=100  TunerSelectOption=Transfer Function Based (PID Tuner App)  InitialConditionSource=internal  InitialConditionForIntegrator=0  InitialConditionForFilter=0  DifferentiatorICPrevScaledInput=0  ExternalReset=none  TrackingMode=off  Kt=1  LimitOutput=off  UpperSaturationLimit=inf  LowerSaturationLimit=-inf  LinearizeAsGain=off  AntiWindupMode=none  Kb=1  POutMin=[]  POutMax=[]  IOutMin=[]  IOutMax=[]  DOutMin=[]  DOutMax=[]  NOutMin=[]  NOutMax=[]  SumOutMin=[]  SumOutMax=[]  SaturationOutMin=[]  SaturationOutMax=[]  PParamMin=[]  PParamMax=[]  IParamMin=[]  IParamMax=[]  DParamMin=[]  DParamMax=[]  NParamMin=[]  NParamMax=[]  KbParamMin=[]  KbParamMax=[]  KtParamMin=[]  KtParamMax=[]  KbOutMin=[]  KbOutMax=[]  KtOutMin=[]  KtOutMax=[]  IntegratorOutMin=[]  IntegratorOutMax=[]  FilterOutMin=[]  FilterOutMax=[]  SumI1OutMin=[]  SumI1OutMax=[]  SumI2OutMin=[]  SumI2OutMax=[]  SumI3OutMin=[]  SumI3OutMax=[]  SumI4OutMin=[]  SumI4OutMax=[]  SumDOutMin=[]  SumDOutMax=[]  DifferentiatorOutMin=[]  DifferentiatorOutMax=[]  FilterDiffOutCoefMin=[]  FilterDiffOutCoefMax=[]  ReciprocalOutMin=[]  ReciprocalOutMax=[]  SumDenOutMin=[]  SumDenOutMax=[]  SumNumOutMin=[]  SumNumOutMax=[]  DivideOutMin=[]  DivideOutMax=[]  IntegratorContinuousStateAttributes=''  IntegratorStateMustResolveToSignalObject=off  IntegratorRTWStateStorageClass=Auto  FilterContinuousStateAttributes=''  FilterStateMustResolveToSignalObject=off  FilterRTWStateStorageClass=Auto  ParallelPVariant=InternalParameters  IdealPVariant=Disabled  IVariant=InternalParameters  DVariant=InternalParameters  IntegratorVariant=Discrete  SatVariant=Disabled  AWVariant=Passthrough  PCopyVariant=Disabled  TRVariant=Disabled  FdbkBlocksVariant=Forward  IdealPFdbkVariant=Disabled  SatFdbkVariant=Disabled  DerivativeFilterVariant=ForwardEulerFilter  NVariant=InternalParameters  NCopyVariant=Disabled  FilterICVariant=InternalICsFilter  IntegratorICVariant=InternalICs  ExternalResetVariant=Disabled  TRSumVariant=Passthrough  SumFdbkVariant=Disabled  SumVariant=Sum_PID
  Reshape{,1..5} (6 alike) : Reshape
  Sat_maxGeschw : Subsystem
  Sat_sollGeschw : Subsystem
  Segmentregler : Subsystem
  StartPos : Selector  IndexOptions=Index vector (port)  Indices=[1 3]  OutputSizes=1
  Sum{,1..2,6} (4 alike) : Sum  Inputs=|+-
  Sum3 : Sum  Inputs=-+|
  Sum4 : Sum  Inputs=++|
  Sum5 : Sum  Inputs=++|
  Terminator{,1..3} (4 alike) : Terminator
  ZielPos : Selector  IndexOptions=Index vector (port)  Indices=[1 3]  OutputSizes=1
  ZielZeit : Selector  IndexOptions=Index vector (port)  Indices=[1 3]  OutputSizes=1
  maxGeschw : Selector  IndexOptions=Index vector (port)  Indices=[1 3]  OutputSizes=1
  sollGeschw : Selector  IndexOptions=Index vector (port)  Indices=[1 3]  OutputSizes=1
  Überwachung : Subsystem
  Out1 : Outport  VectorParamsAs1DForOutWhenUnconnected=off
  wires:
  [LOG_dynZielZeit] -> Terminator3/1
  Segmentregler/6(dynZielZeit) -> [LOG_dynZielZeit]
  [MvmtPerformance] -> Segmentregler/4(MvmtPerf_lagTime)
  [PAR_isAxis] -> MvmtPerformance/2
  [RUN_MvmtPerformance] -> MvmtPerformance/1
  MvmtPerformance/1 -> Reshape5/1
  Reshape5/1 -> [MvmtPerformance]
  [sollGeschw] -> Überwachung/9(sollGeschw)
  [ticksSinceSegBeginn] -> Überwachung/8(ticksSinceSegBeginn)
  Segmentregler/5(ticksSinceSegBeginn) -> [ticksSinceSegBeginn]
  Überwachung/1(Performance Indicator) -> [perfIndicator]
  Data Store Read1/1 -> Assignment1/1
  [perfIndicator] -> Assignment1/2
  [PAR_isAxis] -> Assignment1/3
  Assignment1/1 -> Data Store Write1/1
  [ZielZeit] -> Überwachung/7(ZielZeit)
  [LOG_prevZielZeit] -> Überwachung/6(prevZielZeit)
  [RestZeit] -> Überwachung/5(RestZeit)
  [LOG_istGeschw] -> Überwachung/4(istGeschw)
  [StartPos] -> Überwachung/3(StartPos)
  [ZielPos] -> Überwachung/2(ZielPos)
  [IstPos] -> Überwachung/1(istPos)
  Constant/1 -> Sum3/1
  Sum3/1 -> Sat_maxGeschw/1(Threshold)
  [maxGeschw] -> Sum3/2
  Segmentregler/4(RestZeit) -> [RestZeit]
  Assignment/1 -> Data Store Write/1
  [PAR_isAxis] -> Assignment/3
  [IstPos] -> Assignment/2
  Data Store Read/1 -> Assignment/1
  Reshape3/1 -> [ZielZeit]
  Reshape4/1 -> [StartPos]
  Reshape2/1 -> [maxGeschw]
  Reshape1/1 -> [sollGeschw]
  Reshape/1 -> [ZielPos]
  [LOG_trigSegmentBeginn] -> Terminator1/1
  [LOG_prevZielZeit] -> Terminator/1
  Segmentregler/3(LOG_istGeschw) -> [LOG_istGeschw]
  Segmentregler/2(LOG_trigSegmentBeginn) -> [LOG_trigSegmentBeginn]
  Segmentregler/1(LOG_prevZielZeit) -> [LOG_prevZielZeit]
  StartPos/1 -> Reshape4/1
  [RUN_StartPos] -> StartPos/1
  [PAR_isAxis] -> StartPos/2
  [PAR_isAxis] -> ZielZeit/2
  [RUN_ZielZeit] -> ZielZeit/1
  ZielZeit/1 -> Reshape3/1
  maxGeschw/1 -> Reshape2/1
  [RUN_maxGeschw] -> maxGeschw/1
  [PAR_isAxis] -> maxGeschw/2
  [PAR_isAxis] -> sollGeschw/2
  [RUN_sollGeschw] -> sollGeschw/1
  sollGeschw/1 -> Reshape1/1
  ZielPos/1 -> Reshape/1
  [RUN_ZielPos] -> ZielPos/1
  [PAR_isAxis] -> ZielPos/2
  PAR_isAxis/1 -> [PAR_isAxis]
  [sollGeschw] -> Sat_sollGeschw/1(Threshold)
  [sollGeschw] -> Segmentregler/3(Sollgeschw)
  [StartPos] -> Sum6/2
  [StartPos] -> Sum5/1
  Segmentregler/7(Output) -> Sum4/1
  [IstPos] -> Segmentregler/2(Achse_Pos)
  [ZielZeit] -> Segmentregler/1(Zielzeit)
  [ZielPos] -> Sum6/1
  Sum5/1 -> Out1/1
  Discrete-Time Integrator1/1 -> Sum/2, Sum5/2, [IstPos]
  Sat_maxGeschw/1(Out) -> Sum2/1
  PID_2/1 -> Sum1/1
  Sum1/1 -> PID_3/1
  Discrete-Time Integrator/1 -> [currVel], Sum2/2, Discrete-Time Integrator1/1
  Sum6/1 -> Sum/1
  Sum2/1 -> PID_2/1
  Discrete Transfer Fcn/1 -> Sum1/2, Discrete-Time Integrator/1
  PID_3/1 -> Discrete Transfer Fcn/1
  Sum4/1 -> Sat_maxGeschw/2(In)
  Sat_sollGeschw/1(Out) -> Sum4/2
  PID_1/1 -> Sat_sollGeschw/2(In)
  Sum/1 -> PID_1/1, Segmentregler/5(Regelfehler Pos)
  [LOG_istGeschw] -> Terminator2/1
  Assignment2/1 -> Data Store Write2/1
  Data Store Read2/1 -> Assignment2/1
  [PAR_isAxis] -> Assignment2/3
  [currVel] -> Assignment2/2

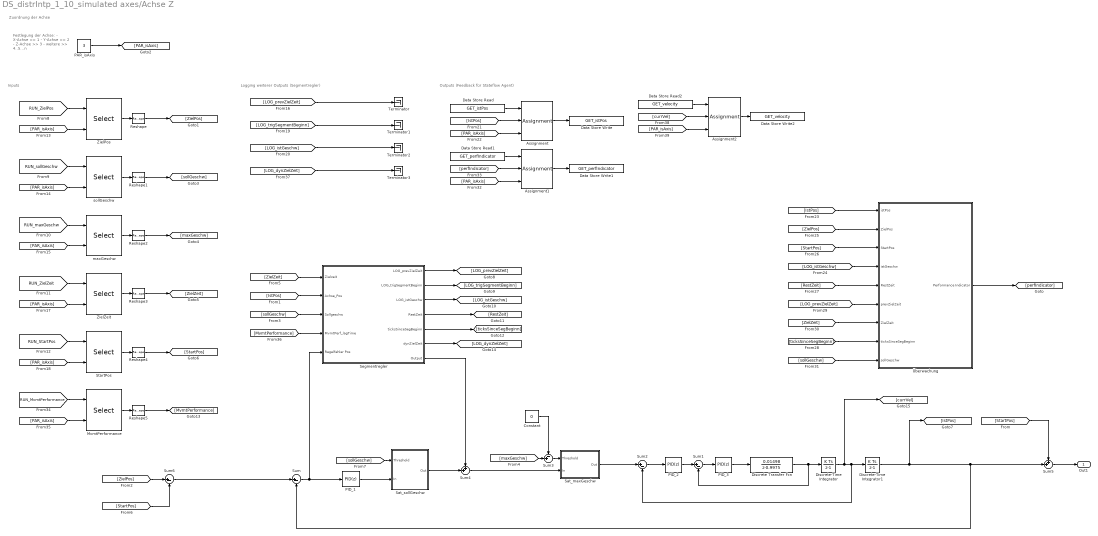
== system DS_distrIntp_1_10_simulated axes/Achse Z ==
  note: Outputs (Feedback für Stateflow Agent)
  note: Logging weiterer Outputs (Segmentregler)
  note: Zuordnung der Achse
  note: Festlegung der Achse:
      | - X-Achse >> 1
      | - Y-Achse >> 2
      | - Z-Achse >> 3
      | - weitere >> 4..5...n
  note: Inputs
  Assignment : Assignment  DiagnosticForDimensions=Warning  IndexOptions=Index vector (port)  Indices=1  OutputSizes=1
  Assignment1 : Assignment  DiagnosticForDimensions=Warning  IndexOptions=Index vector (port)  Indices=1  OutputSizes=1
  Assignment2 : Assignment  DiagnosticForDimensions=Warning  IndexOptions=Index vector (port)  Indices=1  OutputSizes=1
  Constant : Constant  Value=0
  Data Store Read : DataStoreRead  DataStoreName=GET_istPos
  Data Store Read1 : DataStoreRead  DataStoreName=GET_perfIndicator
  Data Store Read2 : DataStoreRead  DataStoreName=GET_velocity
  Data Store Write : DataStoreWrite  DataStoreName=GET_istPos
  Data Store Write1 : DataStoreWrite  DataStoreName=GET_perfIndicator
  Data Store Write2 : DataStoreWrite  DataStoreName=GET_velocity
  Discrete Transfer Fcn : DiscreteTransferFcn  Numerator=0.01498  Denominator=[1 -0.9975]
  Discrete-Time Integrator : DiscreteIntegrator  SampleTime=-1  ICPrevOutput=DiscIntNeverNeededParam  ICPrevScaledInput=DiscIntNeverNeededParam
  Discrete-Time Integrator1 : DiscreteIntegrator  SampleTime=-1  ICPrevOutput=DiscIntNeverNeededParam  ICPrevScaledInput=DiscIntNeverNeededParam
  MvmtPerformance : Selector  IndexOptions=Index vector (port)  Indices=[1 3]  OutputSizes=1
  PAR_isAxis : Constant  Value=3
  PID_1 : simulink/Continuous/PID Controller  Controller=PID  Form=Parallel  TimeDomain=Discrete-time  SampleTime=-1  IntegratorMethod=Forward Euler  FilterMethod=Forward Euler  ControllerParametersSource=internal  P=20  I=0  D=0  UseFilter=on  N=100  TunerSelectOption=Transfer Function Based (PID Tuner App)  InitialConditionSource=internal  InitialConditionForIntegrator=0  InitialConditionForFilter=0  DifferentiatorICPrevScaledInput=0  ExternalReset=none  TrackingMode=off  Kt=1  LimitOutput=off  UpperSaturationLimit=inf  LowerSaturationLimit=-inf  LinearizeAsGain=off  AntiWindupMode=none  Kb=1  POutMin=[]  POutMax=[]  IOutMin=[]  IOutMax=[]  DOutMin=[]  DOutMax=[]  NOutMin=[]  NOutMax=[]  SumOutMin=[]  SumOutMax=[]  SaturationOutMin=[]  SaturationOutMax=[]  PParamMin=[]  PParamMax=[]  IParamMin=[]  IParamMax=[]  DParamMin=[]  DParamMax=[]  NParamMin=[]  NParamMax=[]  KbParamMin=[]  KbParamMax=[]  KtParamMin=[]  KtParamMax=[]  KbOutMin=[]  KbOutMax=[]  KtOutMin=[]  KtOutMax=[]  IntegratorOutMin=[]  IntegratorOutMax=[]  FilterOutMin=[]  FilterOutMax=[]  SumI1OutMin=[]  SumI1OutMax=[]  SumI2OutMin=[]  SumI2OutMax=[]  SumI3OutMin=[]  SumI3OutMax=[]  SumI4OutMin=[]  SumI4OutMax=[]  SumDOutMin=[]  SumDOutMax=[]  DifferentiatorOutMin=[]  DifferentiatorOutMax=[]  FilterDiffOutCoefMin=[]  FilterDiffOutCoefMax=[]  ReciprocalOutMin=[]  ReciprocalOutMax=[]  SumDenOutMin=[]  SumDenOutMax=[]  SumNumOutMin=[]  SumNumOutMax=[]  DivideOutMin=[]  DivideOutMax=[]  IntegratorContinuousStateAttributes=''  IntegratorStateMustResolveToSignalObject=off  IntegratorRTWStateStorageClass=Auto  FilterContinuousStateAttributes=''  FilterStateMustResolveToSignalObject=off  FilterRTWStateStorageClass=Auto  ParallelPVariant=InternalParameters  IdealPVariant=Disabled  IVariant=InternalParameters  DVariant=InternalParameters  IntegratorVariant=Discrete  SatVariant=Disabled  AWVariant=Passthrough  PCopyVariant=Disabled  TRVariant=Disabled  FdbkBlocksVariant=Forward  IdealPFdbkVariant=Disabled  SatFdbkVariant=Disabled  DerivativeFilterVariant=ForwardEulerFilter  NVariant=InternalParameters  NCopyVariant=Disabled  FilterICVariant=InternalICsFilter  IntegratorICVariant=InternalICs  ExternalResetVariant=Disabled  TRSumVariant=Passthrough  SumFdbkVariant=Disabled  SumVariant=Sum_PID
  PID_2 : simulink/Continuous/PID Controller  Controller=PID  Form=Parallel  TimeDomain=Discrete-time  SampleTime=-1  IntegratorMethod=Forward Euler  FilterMethod=Forward Euler  ControllerParametersSource=internal  P=20  I=1  D=0  UseFilter=on  N=100  TunerSelectOption=Transfer Function Based (PID Tuner App)  InitialConditionSource=internal  InitialConditionForIntegrator=0  InitialConditionForFilter=0  DifferentiatorICPrevScaledInput=0  ExternalReset=none  TrackingMode=off  Kt=1  LimitOutput=off  UpperSaturationLimit=inf  LowerSaturationLimit=-inf  LinearizeAsGain=off  AntiWindupMode=none  Kb=1  POutMin=[]  POutMax=[]  IOutMin=[]  IOutMax=[]  DOutMin=[]  DOutMax=[]  NOutMin=[]  NOutMax=[]  SumOutMin=[]  SumOutMax=[]  SaturationOutMin=[]  SaturationOutMax=[]  PParamMin=[]  PParamMax=[]  IParamMin=[]  IParamMax=[]  DParamMin=[]  DParamMax=[]  NParamMin=[]  NParamMax=[]  KbParamMin=[]  KbParamMax=[]  KtParamMin=[]  KtParamMax=[]  KbOutMin=[]  KbOutMax=[]  KtOutMin=[]  KtOutMax=[]  IntegratorOutMin=[]  IntegratorOutMax=[]  FilterOutMin=[]  FilterOutMax=[]  SumI1OutMin=[]  SumI1OutMax=[]  SumI2OutMin=[]  SumI2OutMax=[]  SumI3OutMin=[]  SumI3OutMax=[]  SumI4OutMin=[]  SumI4OutMax=[]  SumDOutMin=[]  SumDOutMax=[]  DifferentiatorOutMin=[]  DifferentiatorOutMax=[]  FilterDiffOutCoefMin=[]  FilterDiffOutCoefMax=[]  ReciprocalOutMin=[]  ReciprocalOutMax=[]  SumDenOutMin=[]  SumDenOutMax=[]  SumNumOutMin=[]  SumNumOutMax=[]  DivideOutMin=[]  DivideOutMax=[]  IntegratorContinuousStateAttributes=''  IntegratorStateMustResolveToSignalObject=off  IntegratorRTWStateStorageClass=Auto  FilterContinuousStateAttributes=''  FilterStateMustResolveToSignalObject=off  FilterRTWStateStorageClass=Auto  ParallelPVariant=InternalParameters  IdealPVariant=Disabled  IVariant=InternalParameters  DVariant=InternalParameters  IntegratorVariant=Discrete  SatVariant=Disabled  AWVariant=Passthrough  PCopyVariant=Disabled  TRVariant=Disabled  FdbkBlocksVariant=Forward  IdealPFdbkVariant=Disabled  SatFdbkVariant=Disabled  DerivativeFilterVariant=ForwardEulerFilter  NVariant=InternalParameters  NCopyVariant=Disabled  FilterICVariant=InternalICsFilter  IntegratorICVariant=InternalICs  ExternalResetVariant=Disabled  TRSumVariant=Passthrough  SumFdbkVariant=Disabled  SumVariant=Sum_PID
  PID_3 : simulink/Continuous/PID Controller  Controller=PID  Form=Parallel  TimeDomain=Discrete-time  SampleTime=-1  IntegratorMethod=Forward Euler  FilterMethod=Forward Euler  ControllerParametersSource=internal  P=20  I=1  D=0  UseFilter=on  N=100  TunerSelectOption=Transfer Function Based (PID Tuner App)  InitialConditionSource=internal  InitialConditionForIntegrator=0  InitialConditionForFilter=0  DifferentiatorICPrevScaledInput=0  ExternalReset=none  TrackingMode=off  Kt=1  LimitOutput=off  UpperSaturationLimit=inf  LowerSaturationLimit=-inf  LinearizeAsGain=off  AntiWindupMode=none  Kb=1  POutMin=[]  POutMax=[]  IOutMin=[]  IOutMax=[]  DOutMin=[]  DOutMax=[]  NOutMin=[]  NOutMax=[]  SumOutMin=[]  SumOutMax=[]  SaturationOutMin=[]  SaturationOutMax=[]  PParamMin=[]  PParamMax=[]  IParamMin=[]  IParamMax=[]  DParamMin=[]  DParamMax=[]  NParamMin=[]  NParamMax=[]  KbParamMin=[]  KbParamMax=[]  KtParamMin=[]  KtParamMax=[]  KbOutMin=[]  KbOutMax=[]  KtOutMin=[]  KtOutMax=[]  IntegratorOutMin=[]  IntegratorOutMax=[]  FilterOutMin=[]  FilterOutMax=[]  SumI1OutMin=[]  SumI1OutMax=[]  SumI2OutMin=[]  SumI2OutMax=[]  SumI3OutMin=[]  SumI3OutMax=[]  SumI4OutMin=[]  SumI4OutMax=[]  SumDOutMin=[]  SumDOutMax=[]  DifferentiatorOutMin=[]  DifferentiatorOutMax=[]  FilterDiffOutCoefMin=[]  FilterDiffOutCoefMax=[]  ReciprocalOutMin=[]  ReciprocalOutMax=[]  SumDenOutMin=[]  SumDenOutMax=[]  SumNumOutMin=[]  SumNumOutMax=[]  DivideOutMin=[]  DivideOutMax=[]  IntegratorContinuousStateAttributes=''  IntegratorStateMustResolveToSignalObject=off  IntegratorRTWStateStorageClass=Auto  FilterContinuousStateAttributes=''  FilterStateMustResolveToSignalObject=off  FilterRTWStateStorageClass=Auto  ParallelPVariant=InternalParameters  IdealPVariant=Disabled  IVariant=InternalParameters  DVariant=InternalParameters  IntegratorVariant=Discrete  SatVariant=Disabled  AWVariant=Passthrough  PCopyVariant=Disabled  TRVariant=Disabled  FdbkBlocksVariant=Forward  IdealPFdbkVariant=Disabled  SatFdbkVariant=Disabled  DerivativeFilterVariant=ForwardEulerFilter  NVariant=InternalParameters  NCopyVariant=Disabled  FilterICVariant=InternalICsFilter  IntegratorICVariant=InternalICs  ExternalResetVariant=Disabled  TRSumVariant=Passthrough  SumFdbkVariant=Disabled  SumVariant=Sum_PID
  Reshape{,1..5} (6 alike) : Reshape
  Sat_maxGeschw : Subsystem
  Sat_sollGeschw : Subsystem
  Segmentregler : Subsystem
  StartPos : Selector  IndexOptions=Index vector (port)  Indices=[1 3]  OutputSizes=1
  Sum{,1..2,6} (4 alike) : Sum  Inputs=|+-
  Sum3 : Sum  Inputs=-+|
  Sum4 : Sum  Inputs=++|
  Sum5 : Sum  Inputs=++|
  Terminator{,1..3} (4 alike) : Terminator
  ZielPos : Selector  IndexOptions=Index vector (port)  Indices=[1 3]  OutputSizes=1
  ZielZeit : Selector  IndexOptions=Index vector (port)  Indices=[1 3]  OutputSizes=1
  maxGeschw : Selector  IndexOptions=Index vector (port)  Indices=[1 3]  OutputSizes=1
  sollGeschw : Selector  IndexOptions=Index vector (port)  Indices=[1 3]  OutputSizes=1
  Überwachung : Subsystem
  Out1 : Outport  VectorParamsAs1DForOutWhenUnconnected=off
  wires:
  Sum/1 -> Segmentregler/5(Regelfehler Pos), PID_1/1
  PID_1/1 -> Sat_sollGeschw/2(In)
  Sat_sollGeschw/1(Out) -> Sum4/2
  Sum4/1 -> Sat_maxGeschw/2(In)
  PID_3/1 -> Discrete Transfer Fcn/1
  Discrete Transfer Fcn/1 -> Discrete-Time Integrator/1, Sum1/2
  Sum2/1 -> PID_2/1
  Sum6/1 -> Sum/1
  Discrete-Time Integrator/1 -> [currVel], Discrete-Time Integrator1/1, Sum2/2
  Sum1/1 -> PID_3/1
  PID_2/1 -> Sum1/1
  Sat_maxGeschw/1(Out) -> Sum2/1
  Discrete-Time Integrator1/1 -> [IstPos], Sum5/2, Sum/2
  Sum5/1 -> Out1/1
  [ZielPos] -> Sum6/1
  [ZielZeit] -> Segmentregler/1(Zielzeit)
  [IstPos] -> Segmentregler/2(Achse_Pos)
  Segmentregler/7(Output) -> Sum4/1
  [StartPos] -> Sum5/1
  [StartPos] -> Sum6/2
  [sollGeschw] -> Segmentregler/3(Sollgeschw)
  [sollGeschw] -> Sat_sollGeschw/1(Threshold)
  PAR_isAxis/1 -> [PAR_isAxis]
  [PAR_isAxis] -> ZielPos/2
  [RUN_ZielPos] -> ZielPos/1
  ZielPos/1 -> Reshape/1
  sollGeschw/1 -> Reshape1/1
  [RUN_sollGeschw] -> sollGeschw/1
  [PAR_isAxis] -> sollGeschw/2
  [PAR_isAxis] -> maxGeschw/2
  [RUN_maxGeschw] -> maxGeschw/1
  maxGeschw/1 -> Reshape2/1
  ZielZeit/1 -> Reshape3/1
  [RUN_ZielZeit] -> ZielZeit/1
  [PAR_isAxis] -> ZielZeit/2
  [PAR_isAxis] -> StartPos/2
  [RUN_StartPos] -> StartPos/1
  StartPos/1 -> Reshape4/1
  Segmentregler/1(LOG_prevZielZeit) -> [LOG_prevZielZeit]
  Segmentregler/2(LOG_trigSegmentBeginn) -> [LOG_trigSegmentBeginn]
  Segmentregler/3(LOG_istGeschw) -> [LOG_istGeschw]
  [LOG_prevZielZeit] -> Terminator/1
  [LOG_trigSegmentBeginn] -> Terminator1/1
  Reshape/1 -> [ZielPos]
  Reshape1/1 -> [sollGeschw]
  Reshape2/1 -> [maxGeschw]
  Reshape4/1 -> [StartPos]
  Reshape3/1 -> [ZielZeit]
  Data Store Read/1 -> Assignment/1
  [IstPos] -> Assignment/2
  [PAR_isAxis] -> Assignment/3
  Assignment/1 -> Data Store Write/1
  Segmentregler/4(RestZeit) -> [RestZeit]
  [maxGeschw] -> Sum3/2
  Sum3/1 -> Sat_maxGeschw/1(Threshold)
  Constant/1 -> Sum3/1
  [IstPos] -> Überwachung/1(istPos)
  [ZielPos] -> Überwachung/2(ZielPos)
  [StartPos] -> Überwachung/3(StartPos)
  [LOG_istGeschw] -> Überwachung/4(istGeschw)
  [RestZeit] -> Überwachung/5(RestZeit)
  [LOG_prevZielZeit] -> Überwachung/6(prevZielZeit)
  [ZielZeit] -> Überwachung/7(ZielZeit)
  Assignment1/1 -> Data Store Write1/1
  [PAR_isAxis] -> Assignment1/3
  [perfIndicator] -> Assignment1/2
  Data Store Read1/1 -> Assignment1/1
  Überwachung/1(Performance Indicator) -> [perfIndicator]
  Segmentregler/5(ticksSinceSegBeginn) -> [ticksSinceSegBeginn]
  [ticksSinceSegBeginn] -> Überwachung/8(ticksSinceSegBeginn)
  [sollGeschw] -> Überwachung/9(sollGeschw)
  Reshape5/1 -> [MvmtPerformance]
  MvmtPerformance/1 -> Reshape5/1
  [RUN_MvmtPerformance] -> MvmtPerformance/1
  [PAR_isAxis] -> MvmtPerformance/2
  [MvmtPerformance] -> Segmentregler/4(MvmtPerf_lagTime)
  Segmentregler/6(dynZielZeit) -> [LOG_dynZielZeit]
  [LOG_dynZielZeit] -> Terminator3/1
  [LOG_istGeschw] -> Terminator2/1
  Assignment2/1 -> Data Store Write2/1
  Data Store Read2/1 -> Assignment2/1
  [PAR_isAxis] -> Assignment2/3
  [currVel] -> Assignment2/2
